simulink model "Environment"  (R2015a)
settings: Solver=FixedStepDiscrete  StartTime=0.0  StopTime=10.0  FixedStep=delta_t  RelTol=1e-3
settings Model: Creator=Kerianne  LastModifiedBy=Kerianne
settings DataIOCC: SaveFormat=Structure
settings OptimizationCC: InlineParams=on  ExpressionDepthLimit=2147483647
settings DebuggingCC: UnderspecifiedInitializationDetection=Classic  MergeDetectMultiDrivingBlocksExec=none  SolverPrmCheckMsg=warning  StateNameClashWarn=warning

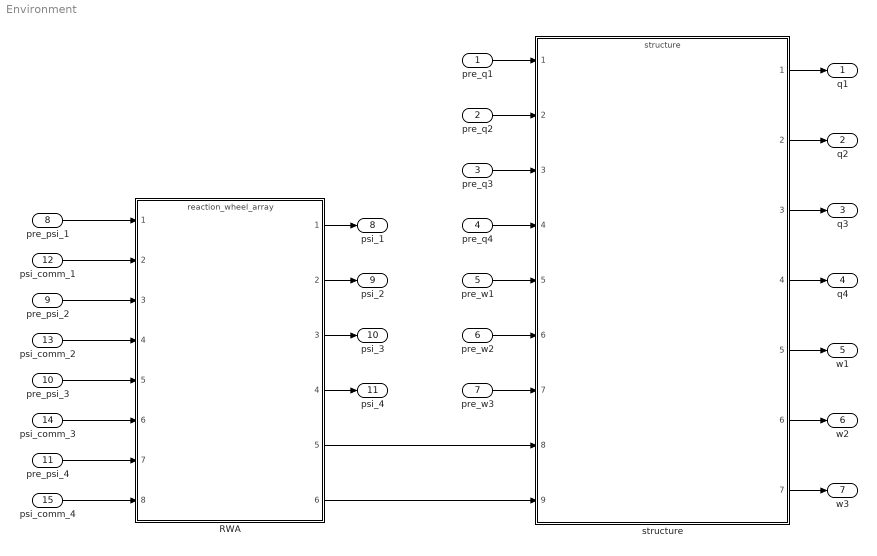
== system Environment ==
  pre_q1 : Inport
  pre_q2 : Inport  Port=2
  pre_q3 : Inport  Port=3
  pre_q4 : Inport  Port=4
  pre_w1 : Inport  Port=5
  pre_w2 : Inport  Port=6
  pre_w3 : Inport  Port=7
  pre_psi_1 : Inport  Port=8
  pre_psi_2 : Inport  Port=9
  pre_psi_3 : Inport  Port=10
  pre_psi_4 : Inport  Port=11
  "psi_comm_1 " : Inport  Port=12
  psi_comm_2 : Inport  Port=13
  psi_comm_3 : Inport  Port=14
  psi_comm_4 : Inport  Port=15
  RWA : ModelReference  ModelNameDialog=reaction_wheel_array  SimulationMode=Normal  ModelReferenceVersion=1.15  CopyOfModelName=reaction_wheel_array  DefaultDataLogging=on
  structure : ModelReference  ModelNameDialog=structure  SimulationMode=Normal  ModelReferenceVersion=1.25  CopyOfModelName=structure  DefaultDataLogging=on
  q1 : Outport
  q2 : Outport  Port=2
  q3 : Outport  Port=3
  q4 : Outport  Port=4
  w1 : Outport  Port=5
  w2 : Outport  Port=6
  w3 : Outport  Port=7
  psi_1 : Outport  Port=8
  psi_2 : Outport  Port=9
  psi_3 : Outport  Port=10
  psi_4 : Outport  Port=11
  wires:
  pre_psi_1/1 -> RWA/1
  "psi_comm_1 "/1 -> RWA/2
  pre_psi_2/1 -> RWA/3
  psi_comm_2/1 -> RWA/4
  pre_psi_3/1 -> RWA/5
  psi_comm_3/1 -> RWA/6
  structure/7 -> w3/1
  structure/6 -> w2/1
  structure/5 -> w1/1
  structure/4 -> q4/1
  structure/3 -> q3/1
  structure/2 -> q2/1
  structure/1 -> q1/1
  pre_w3/1 -> structure/7
  pre_w2/1 -> structure/6
  pre_w1/1 -> structure/5
  pre_q4/1 -> structure/4
  pre_q3/1 -> structure/3
  pre_q2/1 -> structure/2
  pre_q1/1 -> structure/1
  RWA/3 -> psi_3/1
  RWA/2 -> psi_2/1
  RWA/1 -> psi_1/1
  RWA/6 -> structure/9
  RWA/5 -> structure/8
  RWA/4 -> psi_4/1
  pre_psi_4/1 -> RWA/7
  psi_comm_4/1 -> RWA/8
